simulink model "sFunction_Sims"  (R2023b)
settings: Solver=ode3  StartTime=0.0  StopTime=30  FixedStep=0.01  RelTol=1e-3
settings Model: Creator=erdem  LastModifiedBy=erdem

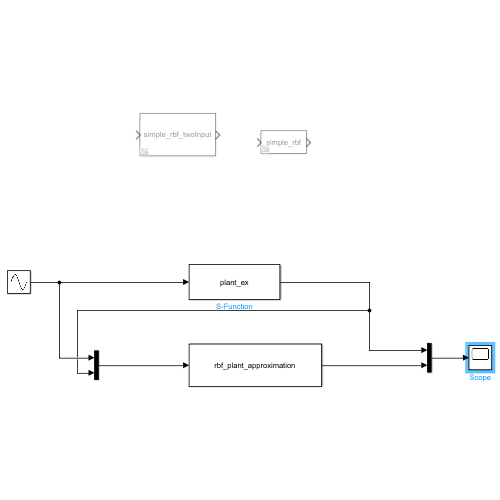
[thumbnail: Simulink's stored preview of the top-level diagram]
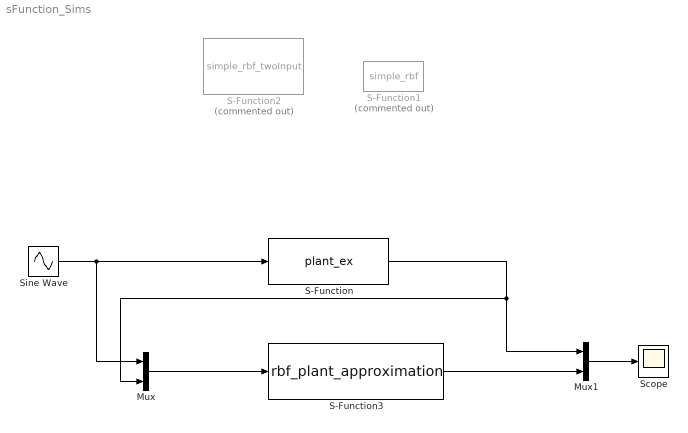
== system sFunction_Sims ==
  Mux : Mux  Inputs=2
  Mux1 : Mux  Inputs=2
  S-Function : S-Function  FunctionName=plant_ex  SFunctionDeploymentMode=off  EnableBusSupport=off
  S-Function1 : S-Function  Commented=on  FunctionName=simple_rbf  SFunctionDeploymentMode=off  EnableBusSupport=off
  S-Function2 : S-Function  Commented=on  FunctionName=simple_rbf_twoInput  SFunctionDeploymentMode=off  EnableBusSupport=off
  S-Function3 : S-Function  FunctionName=rbf_plant_approximation  SFunctionDeploymentMode=off  EnableBusSupport=off
  Scope : Scope
  Sine Wave : Sin  SampleTime=0
  wires:
  Sine Wave/1 -> Mux/1, S-Function/1
  Mux/1 -> S-Function3/1
  S-Function/1 -> Mux/2, Mux1/1
  S-Function3/1 -> Mux1/2
  Mux1/1 -> Scope/1
